simulink model "FullWaveRect"  (R2015a)
settings: Solver=ode23t  StartTime=0.0  StopTime=0.05  RelTol=1e-6
libraries: powerlib x12, powerlib_meascontrol x1
settings Model: Creator=asus  LastModifiedBy=asus
settings SolverCC: ZeroCrossControl=DisableAll  ZeroCrossAlgorithm=Adaptive

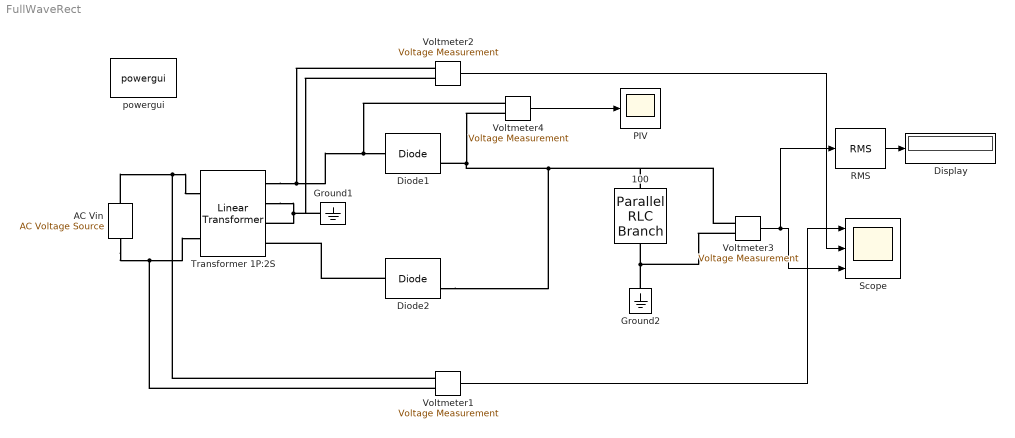
== system FullWaveRect ==
  "100 " : powerlib/Elements/Parallel RLC Branch  LConnTagsString=a  RConnTagsString=__new0  BranchType=R  Resistance=100  Inductance=1e-3  SetiL0=off  InitialCurrent=0  Capacitance=100e-6  Setx0=off  InitialVoltage=0  Measurements=None
  AC Vin : powerlib/Electrical Sources/AC Voltage Source  Amplitude=220*sqrt(2)  Phase=0  Frequency=60  SampleTime=0  Measurements=None
  Diode1 : powerlib/Power Electronics/Diode  Ron=0.001  Lon=0  Vf=0.8  IC=0  UseSnubber=off  Rs=0  Cs=0  Measurements=on
  Diode2 : powerlib/Power Electronics/Diode  Ron=0.001  Lon=0  Vf=0.8  IC=0  UseSnubber=off  Rs=0  Cs=0  Measurements=on
  Display : Display
  Ground1 : powerlib/Elements/Ground  LConnTagsString=a
  Ground2 : powerlib/Elements/Ground  LConnTagsString=a
  PIV : Scope
      settings: TimeRange=0.04999000000000001  YMin=-20  YMax=20
  RMS : powerlib_meascontrol/Measurements/RMS  TrueRMS=on  Freq=60  RMSInit=120  Ts=0
  Scope : Scope  NumInputPorts=3
      settings: TimeRange=0.04999000000000001  YMin=-20~-20~13  YMax=20~20~15
  Transformer 1P:2S : powerlib/Elements/Linear Transformer  UNITS=SI  NominalPower=[ 250e6 60 ]  winding1=[220 0 0]  winding2=[12 0 0]  ThreeWindings=on  winding3=[12 0 0]  RmLm=[inf inf]  Measurements=None  DataType=on
  Voltmeter{1..4} (4 alike) : powerlib/Measurements/Voltage Measurement  PhasorSimulation=off  OutputType=Complex  PSBequivalent=0
  powergui : powerlib/powergui  Priority=1  SimulationMode=Discrete  SolverType=Tustin/Backward Euler (TBE)  SampleTime=10e-6  frequency=60  SPID=off  DisableSnubberDevices=off  DisableRonSwitches=off  DisableVfSwitches=off  SwTol=0  DisplayEquations=off  Interpol=off  methode=off  Ts=100  FunctionMessages=off  echomessages=off  HookPort=off  EnableUseOfTLC=off  x0status=blocks  frequencyindice=60  Pbase=100e6  ErrMax=1e-4  Iterations=50  UnitsV=kV  UnitsW=MW  buscounter=0  RestoreLinks=warning  ResistiveCurrentMeasurement=off  Frange=[0:2:500]  Ylog=off  Xlog=on  ShowGrid=off  save=off  variable=ZData  structure=0  ZoomFFT=off  StartTime=0.0  cycles=1  DisplayStyle=1  fundamental=60  FreqAxis=off  MaxFrequency=1000  frequencyindicesteady=1  RmsSteady=1  display=off
  wires:
  Voltmeter2/1 -> Scope/2
  Voltmeter1/1 -> Scope/1
  RMS/1 -> Display/1
  Voltmeter3/1 -> RMS/1, Scope/3
  Voltmeter4/1 -> PIV/1
  connections:
  Transformer 1P:2S/RConn2 -- Voltmeter2/LConn2 -- Ground1/LConn1 -- Transformer 1P:2S/RConn3
  Diode2/LConn1 -- Transformer 1P:2S/RConn4
  Transformer 1P:2S/RConn1 -- Voltmeter2/LConn1 -- Voltmeter4/LConn1 -- Diode1/LConn1
  Ground2/LConn1 -- Voltmeter3/LConn2 -- "100 "/RConn1
  AC Vin/RConn1 -- Voltmeter1/LConn1 -- Transformer 1P:2S/LConn1
  AC Vin/LConn1 -- Voltmeter1/LConn2 -- Transformer 1P:2S/LConn2
  Diode2/RConn1 -- Voltmeter3/LConn1 -- "100 "/LConn1 -- Voltmeter4/LConn2 -- Diode1/RConn1
